simulink subsystem "rss_GDVltgLoLvl1Dia"  (R2023a)
settings: Solver=VariableStepAuto  StartTime=0.0  StopTime=10.0  RelTol=1e-3
undefined symbols (not defined in the file): ENM_TYPE_FALT, Gu16_ctGDVltgLoLvl1ConfCnt_C, Gu16_ctGDVltgLoLvl1RcvyCnt_C, Gu16_uGDVltgLoLvl1ConfTrs_C, Gu16_uGDVltgLoLvl1RcvyTrs_C
libraries: vhit_control_library x1, lib_debounce x1, lib_fault_definiteness x1
settings Model: Creator=xiaoqiang.yuan  LastModifiedBy=xiaoqiang.yuan

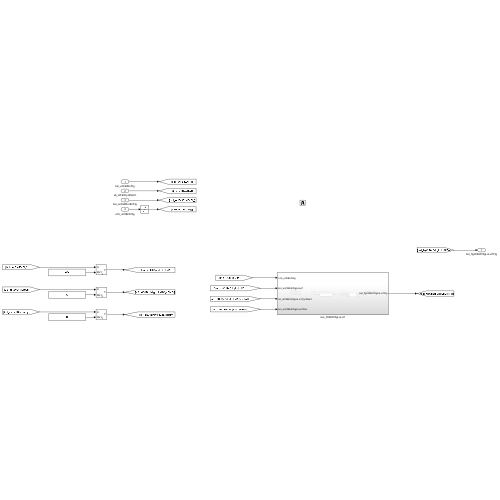
[thumbnail: Simulink's stored preview of the top-level diagram]
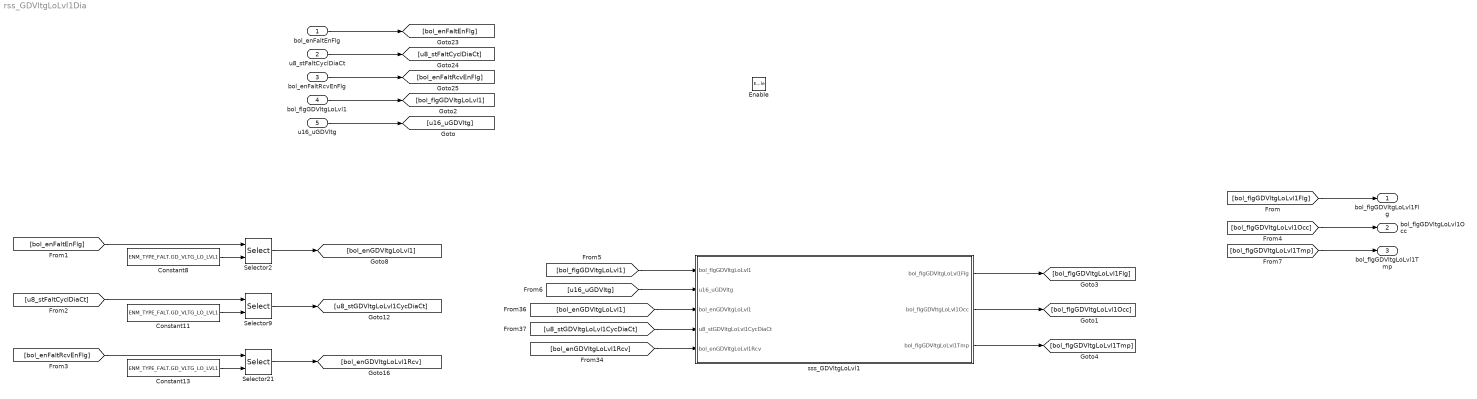
== system rss_GDVltgLoLvl1Dia ==
  bol_enFaltEnFlg : Inport  OutDataTypeStr=boolean
  u8_stFaltCyclDiaCt : Inport  Port=2  OutDataTypeStr=uint8
  bol_enFaltRcvEnFlg : Inport  Port=3  OutDataTypeStr=boolean
  bol_flgGDVltgLoLvl1 : Inport  Port=4  OutDataTypeStr=boolean
  u16_uGDVltg : Inport  Port=5  OutDataTypeStr=dt_Standardize_u16p15b0
  Enable : EnablePort
  Constant11 : Constant  Value=ENM_TYPE_FALT.GD_VLTG_LO_LVL1
  Constant13 : Constant  Value=ENM_TYPE_FALT.GD_VLTG_LO_LVL1
  Constant8 : Constant  Value=ENM_TYPE_FALT.GD_VLTG_LO_LVL1
  Selector2 : Selector  IndexMode=Zero-based  InputPortWidth=Cdbl_numFaltDiaNum  IndexOptions=Index vector (port)  Indices=[1 3]  OutputSizes=1
  Selector21 : Selector  IndexMode=Zero-based  InputPortWidth=Cdbl_numFaltDiaNum  IndexOptions=Index vector (port)  Indices=[1 3]  OutputSizes=1
  Selector9 : Selector  IndexMode=Zero-based  InputPortWidth=Cdbl_numFaltDiaNum  IndexOptions=Index vector (port)  Indices=[1 3]  OutputSizes=1
  sss_GDVltgLoLvl1 : Subsystem
  bol_flgGDVltgLoLvl1Flg : Outport  OutDataTypeStr=boolean
  bol_flgGDVltgLoLvl1Occ : Outport  Port=2  OutDataTypeStr=boolean
  bol_flgGDVltgLoLvl1Tmp : Outport  Port=3  OutDataTypeStr=boolean
  wires:
  [bol_flgGDVltgLoLvl1Flg] -> bol_flgGDVltgLoLvl1Flg/1
  [bol_flgGDVltgLoLvl1] -> sss_GDVltgLoLvl1/1(bol_flgGDVltgLoLvl1)
  [u8_stGDVltgLoLvl1CycDiaCt] -> sss_GDVltgLoLvl1/4(u8_stGDVltgLoLvl1CycDiaCt)
  [bol_enGDVltgLoLvl1] -> sss_GDVltgLoLvl1/3(bol_enGDVltgLoLvl1)
  sss_GDVltgLoLvl1/1(bol_flgGDVltgLoLvl1Flg) -> [bol_flgGDVltgLoLvl1Flg]
  [bol_enGDVltgLoLvl1Rcv] -> sss_GDVltgLoLvl1/5(bol_enGDVltgLoLvl1Rcv)
  u8_stFaltCyclDiaCt/1 -> [u8_stFaltCyclDiaCt]
  bol_enFaltRcvEnFlg/1 -> [bol_enFaltRcvEnFlg]
  bol_enFaltEnFlg/1 -> [bol_enFaltEnFlg]
  [u8_stFaltCyclDiaCt] -> Selector9/1
  [bol_enFaltRcvEnFlg] -> Selector21/1
  [bol_enFaltEnFlg] -> Selector2/1
  Selector21/1 -> [bol_enGDVltgLoLvl1Rcv]
  Selector9/1 -> [u8_stGDVltgLoLvl1CycDiaCt]
  Selector2/1 -> [bol_enGDVltgLoLvl1]
  Constant11/1 -> Selector9/2
  Constant13/1 -> Selector21/2
  Constant8/1 -> Selector2/2
  sss_GDVltgLoLvl1/2(bol_flgGDVltgLoLvl1Occ) -> [bol_flgGDVltgLoLvl1Occ]
  [bol_flgGDVltgLoLvl1Occ] -> bol_flgGDVltgLoLvl1Occ/1
  bol_flgGDVltgLoLvl1/1 -> [bol_flgGDVltgLoLvl1]
  [u16_uGDVltg] -> sss_GDVltgLoLvl1/2(u16_uGDVltg)
  u16_uGDVltg/1 -> [u16_uGDVltg]
  [bol_flgGDVltgLoLvl1Tmp] -> bol_flgGDVltgLoLvl1Tmp/1
  sss_GDVltgLoLvl1/3(bol_flgGDVltgLoLvl1Tmp) -> [bol_flgGDVltgLoLvl1Tmp]

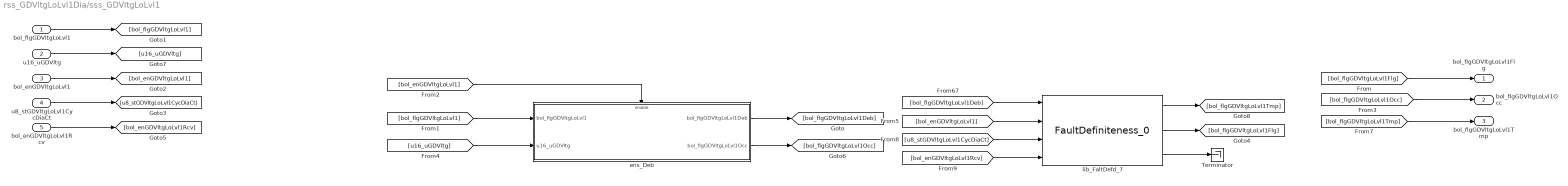
== system rss_GDVltgLoLvl1Dia/sss_GDVltgLoLvl1 ==
  bol_flgGDVltgLoLvl1 : Inport
  u16_uGDVltg : Inport  Port=2
  bol_enGDVltgLoLvl1 : Inport  Port=3
  u8_stGDVltgLoLvl1CycDiaCt : Inport  Port=4
  bol_enGDVltgLoLvl1Rcv : Inport  Port=5
  Terminator : Terminator
  ens_Deb : Subsystem  Variant=on  VariantControlMode=label  VariantControl=Choice  LabelModeActiveChoice=GEELY_PROJECT
  lib_FaltDefd_7 : lib_fault_definiteness/FaultDefiniteness_0  lb_FaltWaitRecvCnt=Gu16_ctGDVltgLoLvl1ConfCnt_C
  bol_flgGDVltgLoLvl1Flg : Outport
  bol_flgGDVltgLoLvl1Occ : Outport  Port=2
  bol_flgGDVltgLoLvl1Tmp : Outport  Port=3
  wires:
  [bol_flgGDVltgLoLvl1Tmp] -> bol_flgGDVltgLoLvl1Tmp/1
  u16_uGDVltg/1 -> [u16_uGDVltg]
  [u16_uGDVltg] -> ens_Deb/2(u16_uGDVltg)
  ens_Deb/2(bol_flgGDVltgLoLvl1Occ) -> [bol_flgGDVltgLoLvl1Occ]
  ens_Deb/1(bol_flgGDVltgLoLvl1Deb) -> [bol_flgGDVltgLoLvl1Deb]
  [bol_enGDVltgLoLvl1] -> ens_Deb/Enable
  [bol_flgGDVltgLoLvl1] -> ens_Deb/1(bol_flgGDVltgLoLvl1)
  [bol_flgGDVltgLoLvl1Occ] -> bol_flgGDVltgLoLvl1Occ/1
  lib_FaltDefd_7/1 -> [bol_flgGDVltgLoLvl1Tmp]
  lib_FaltDefd_7/2 -> [bol_flgGDVltgLoLvl1Flg]
  lib_FaltDefd_7/3 -> Terminator/1
  bol_enGDVltgLoLvl1Rcv/1 -> [bol_enGDVltgLoLvl1Rcv]
  u8_stGDVltgLoLvl1CycDiaCt/1 -> [u8_stGDVltgLoLvl1CycDiaCt]
  bol_enGDVltgLoLvl1/1 -> [bol_enGDVltgLoLvl1]
  [bol_flgGDVltgLoLvl1Flg] -> bol_flgGDVltgLoLvl1Flg/1
  bol_flgGDVltgLoLvl1/1 -> [bol_flgGDVltgLoLvl1]
  [bol_enGDVltgLoLvl1Rcv] -> lib_FaltDefd_7/4
  [u8_stGDVltgLoLvl1CycDiaCt] -> lib_FaltDefd_7/3
  [bol_enGDVltgLoLvl1] -> lib_FaltDefd_7/2
  [bol_flgGDVltgLoLvl1Deb] -> lib_FaltDefd_7/1

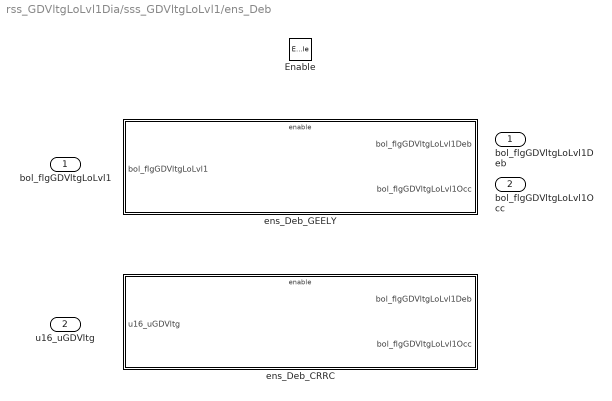
== system rss_GDVltgLoLvl1Dia/sss_GDVltgLoLvl1/ens_Deb ==
  bol_flgGDVltgLoLvl1 : Inport
  u16_uGDVltg : Inport  Port=2
  Enable : EnablePort
  ens_Deb_CRRC : Subsystem  VariantControl=CRRC_PROJECT
  ens_Deb_GEELY : Subsystem  VariantControl=GEELY_PROJECT
  bol_flgGDVltgLoLvl1Deb : Outport
  bol_flgGDVltgLoLvl1Occ : Outport  Port=2

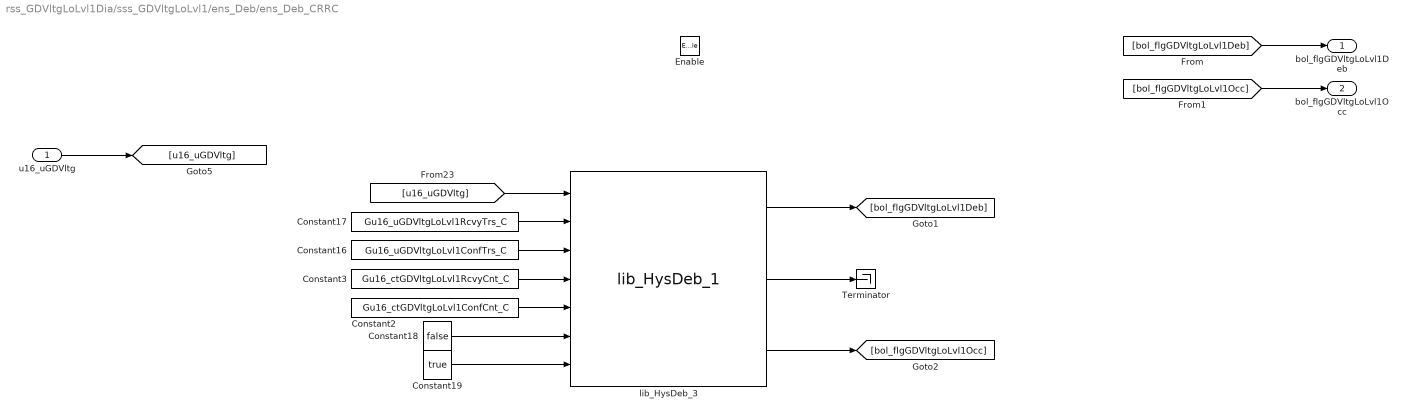
== system rss_GDVltgLoLvl1Dia/sss_GDVltgLoLvl1/ens_Deb/ens_Deb_CRRC ==
  u16_uGDVltg : Inport
  Enable : EnablePort
  Constant16 : Constant  Value=Gu16_uGDVltgLoLvl1ConfTrs_C
  Constant17 : Constant  Value=Gu16_uGDVltgLoLvl1RcvyTrs_C
  Constant18 : Constant  Value=false  OutDataTypeStr=boolean
  Constant19 : Constant  Value=true  OutDataTypeStr=boolean
  Constant2 : Constant  Value=Gu16_ctGDVltgLoLvl1ConfCnt_C
  Constant3 : Constant  Value=Gu16_ctGDVltgLoLvl1RcvyCnt_C
  Terminator : Terminator
  lib_HysDeb_3 : vhit_control_library/lib_HysDeb_1  lb_parInitOutp=0
  bol_flgGDVltgLoLvl1Deb : Outport
  bol_flgGDVltgLoLvl1Occ : Outport  Port=2
  wires:
  [u16_uGDVltg] -> lib_HysDeb_3/1
  Constant16/1 -> lib_HysDeb_3/3
  Constant19/1 -> lib_HysDeb_3/7
  Constant2/1 -> lib_HysDeb_3/5
  lib_HysDeb_3/2 -> Terminator/1
  Constant3/1 -> lib_HysDeb_3/4
  lib_HysDeb_3/1 -> [bol_flgGDVltgLoLvl1Deb]
  Constant18/1 -> lib_HysDeb_3/6
  lib_HysDeb_3/3 -> [bol_flgGDVltgLoLvl1Occ]
  Constant17/1 -> lib_HysDeb_3/2
  [bol_flgGDVltgLoLvl1Deb] -> bol_flgGDVltgLoLvl1Deb/1
  [bol_flgGDVltgLoLvl1Occ] -> bol_flgGDVltgLoLvl1Occ/1
  u16_uGDVltg/1 -> [u16_uGDVltg]

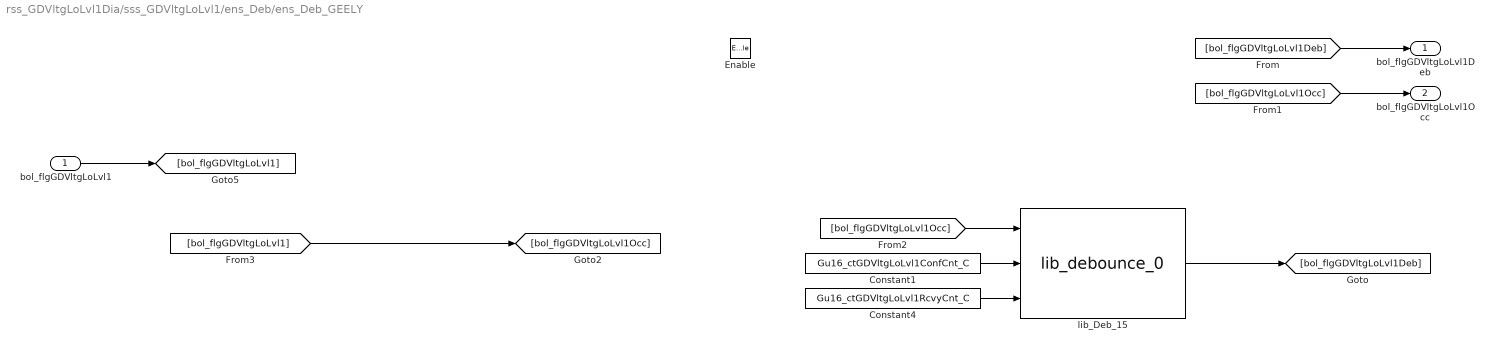
== system rss_GDVltgLoLvl1Dia/sss_GDVltgLoLvl1/ens_Deb/ens_Deb_GEELY ==
  bol_flgGDVltgLoLvl1 : Inport
  Enable : EnablePort
  Constant1 : Constant  Value=Gu16_ctGDVltgLoLvl1ConfCnt_C
  Constant4 : Constant  Value=Gu16_ctGDVltgLoLvl1RcvyCnt_C
  lib_Deb_15 : lib_debounce/lib_debounce_0
  bol_flgGDVltgLoLvl1Deb : Outport
  bol_flgGDVltgLoLvl1Occ : Outport  Port=2
  wires:
  bol_flgGDVltgLoLvl1/1 -> [bol_flgGDVltgLoLvl1]
  [bol_flgGDVltgLoLvl1] -> [bol_flgGDVltgLoLvl1Occ]
  lib_Deb_15/1 -> [bol_flgGDVltgLoLvl1Deb]
  Constant1/1 -> lib_Deb_15/2
  Constant4/1 -> lib_Deb_15/3
  [bol_flgGDVltgLoLvl1Occ] -> lib_Deb_15/1
  [bol_flgGDVltgLoLvl1Occ] -> bol_flgGDVltgLoLvl1Occ/1
  [bol_flgGDVltgLoLvl1Deb] -> bol_flgGDVltgLoLvl1Deb/1
